simulink model "double_integrator"  (R2015b)
settings: Solver=VariableStepAuto  StartTime=0.0  StopTime=10.0  RelTol=1e-3
undefined symbols (not defined in the file): fset, std_R
settings Model: Creator=mgreiff  LastModifiedBy=mgreiff

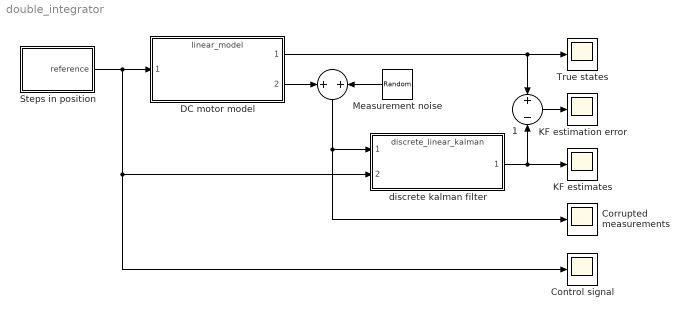
== system double_integrator ==
  " " : Sum  Inputs=+|+
  " 1" : Sum  Inputs=+|-
  Control signal : Scope
  Corrupted measurements : Scope
  DC motor model : ModelReference  ModelNameDialog=linear_model.slx  SimulationMode=Normal  ModelReferenceVersion=1.16  CopyOfModelName=linear_model.slx
  KF estimates : Scope
  KF estimation error : Scope
  Measurement noise : RandomNumber  Mean=std_R.*0  Variance=std_R.^2  SampleTime=fset.h
  Steps in position : Subsystem
  True states : Scope
  discrete kalman filter : ModelReference  ModelNameDialog=discrete_linear_kalman.slx  SimulationMode=Normal  ModelReferenceVersion=1.93  CopyOfModelName=discrete_linear_kalman.slx
  wires:
  DC motor model/1 -> " 1"/1, True states/1
  Steps in position/1(reference) -> Control signal/1, discrete kalman filter/2, DC motor model/1
  Measurement noise/1 -> " "/2
  DC motor model/2 -> " "/1
  " "/1 -> Corrupted measurements/1, discrete kalman filter/1
  discrete kalman filter/1 -> " 1"/2, KF estimates/1
  " 1"/1 -> KF estimation error/1

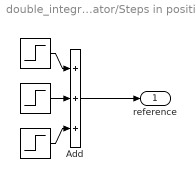
== system double_integrator/Steps in position ==
  "  " : Step  Time=0  SampleTime=0
  "   " : Step  Time=4  After=-2  SampleTime=0
  "    " : Step  Time=8  SampleTime=0
  Add : Sum  Inputs=+++
  reference : Outport
  wires:
  Add/1 -> reference/1
  "   "/1 -> Add/2
  "    "/1 -> Add/3
  "  "/1 -> Add/1
